simulink model "sldemo_counters_2018a"  (R2018a)
settings: Solver=VariableStepAuto  StartTime=0.0  StopTime=600  FixedStep=.01  RelTol=1e-3  AbsTol=1e-6  EnableMultiTasking=on
libraries: simulink x3
Description:
  | Counters Using Conditionally Executed Subsystems
  | 
  | This model shows the contrast between enabled subsystems and triggered
  | subsystems for the same control signal, through the use of counter circuits.
  | After running the simulation, the scope shows three plots.
  | 
  | The first of these plots shows the control signal which is the output of the discrete
  | pulse generator.
  | 
  | The second plot shows the output of the counter circuit in the enabled subsystem.
  | The counter increments while the subsystem is enabled and then holds its output when
  | the subsystem is disabled. The counter resets to zero when the subsystem is re-enabled
  | because the enable port was configured to reset states when enabling.
  | 
  | The third plot shows the output of the counter circuit in the triggered subsystem. The
  | counter increments every rising edge of the control signal.
  | 
  | The signals are shown in a Signal Viewer scope that does not require a scope block to
  | be put into the block diagram.  Instead, the "scope" icon notation on the ports show
  | that a Signal Viewer is attached.  Double click on the scope icon to make the Signal
  | Viewer appear if it is hidden.
settings Model: ModifiedByFormat=The MathWorks, Inc.  EnablePacing=on  PacingRate=30  ExtModeTrigMode=oneshot  ExtModeArmWhenConnect=off  ExtModeAutoUpdateStatusClock=off  Creator=The MathWorks, Inc.  LastModifiedBy=The MathWorks, Inc.
settings SolverCC: AutoScaleAbsTol=off
settings DataIOCC: SaveFormat=Array
settings OptimizationCC: BlockReduction=off  BooleanDataType=off  ExpressionDepthLimit=2147483647  InitFltsAndDblsToZero=on  LifeSpan=inf  BufferReusableBoundary=off
settings DebuggingCC: SaveWithParameterizedLinksMsg=none  SignalResolutionControl=TryResolveAllWithWarning  MultiTaskDSMMsg=warning  MultiTaskCondExecSysMsg=none  IntegerOverflowMsg=none  FcnCallInpInsideContextMsg=warning  BusObjectLabelMismatch=none  StateNameClashWarn=warning  SFUnexpectedBacktrackingDiag=warning  SFNoUnconditionalDefaultTransitionDiag=warning  SFExecutionAtInitializationDiag=none  IntegerSaturationMsg=none
settings HardwareCC: ProdBitPerPointer=32  ProdBitPerSizeT=32  ProdBitPerPtrDiffT=32  ProdLargestAtomicFloat=None  ProdIntDivRoundTo=Undefined  ProdEndianess=Unspecified  ProdWordSize=32  ProdHWDeviceType=32-bit Generic  TargetUnknown=on
settings ModelReferenceCC: PropagateSignalLabelsOutOfModel=off
settings CodeAppCC: StateflowObjectComments=on
settings GRTTargetCC: TargetFcnLib=ansi_tfl_tmw.mat  TargetLangStandard=C89/C90 (ANSI)  CombineOutputUpdateFcns=off  GRTInterface=on
settings ConfigComp: CovMetricSettings=dw  CovSaveCumulativeToWorkspaceVar=on  CovSaveSingleToWorkspaceVar=on  CovExternalEMLEnable=off  CovSFcnEnable=off

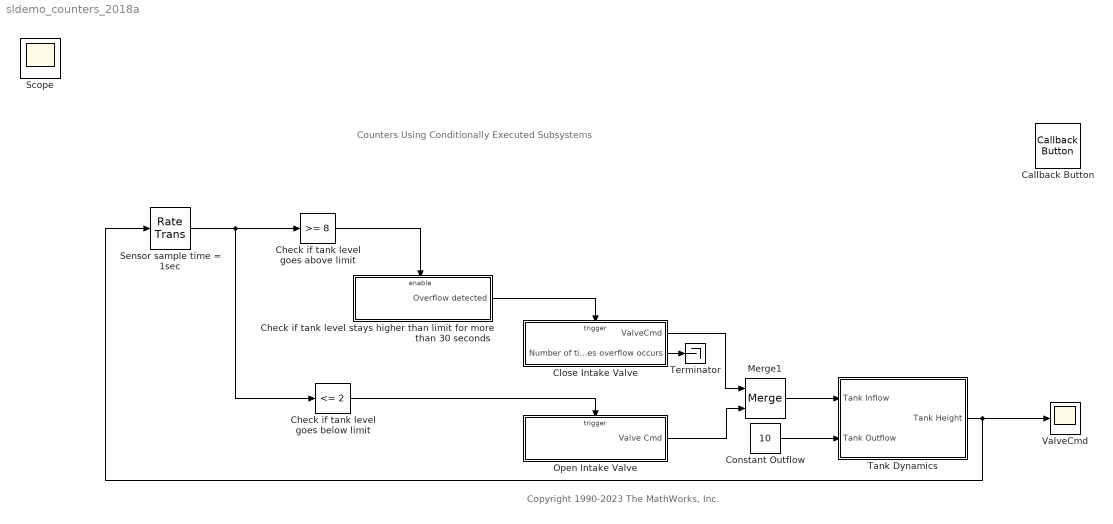
== system sldemo_counters_2018a ==
  note: Counters Using Conditionally Executed Subsystems
  note: Copyright 1990-2023 The MathWorks, Inc.
  Callback Button : CallbackButton  WebBlockId=135  ButtonText=?
      settings: ClickFcn=openExample('simulink_general/sldemo_countersExample')
  Check if tank level goes above limit : simulink/Logic and Bit Operations/Compare To Constant  relop=>=  const=8  OutDataTypeStr=boolean
  Check if tank level goes below limit : simulink/Logic and Bit Operations/Compare To Constant  relop=<=  const=2  OutDataTypeStr=boolean
  Check if tank level stays higher than limit for more than 30 seconds : Subsystem  TreatAsAtomicUnit=on
  Close Intake Valve : Subsystem  TreatAsAtomicUnit=on
  Constant Outflow : Constant  Value=10
  Merge1 : Merge  InitialOutput=2
  Open Intake Valve : Subsystem  TreatAsAtomicUnit=on
  Sensor sample time = 1sec : RateTransition  OutPortSampleTime=1
  Tank Dynamics : Subsystem
  Terminator : Terminator
  ValveCmd : Scope
  Scope : Scope
  wires:
  Close Intake Valve/1(ValveCmd) -> Merge1/1
  Constant Outflow/1 -> Tank Dynamics/2(Tank Outflow)
  Open Intake Valve/1(Valve Cmd) -> Merge1/2
  Check if tank level goes below limit/1 -> Open Intake Valve/Trigger
  Check if tank level stays higher than limit for more than 30 seconds/1(Overflow detected) -> Close Intake Valve/Trigger
  Merge1/1 -> Tank Dynamics/1(Tank Inflow)
  Close Intake Valve/2(Number of times overflow occurs) -> Terminator/1
  Sensor sample time = 1sec/1 -> Check if tank level goes above limit/1, Check if tank level goes below limit/1
  Tank Dynamics/1(Tank Height) -> Sensor sample time = 1sec/1, ValveCmd/1
  Check if tank level goes above limit/1 -> Check if tank level stays higher than limit for more than 30 seconds/Enable

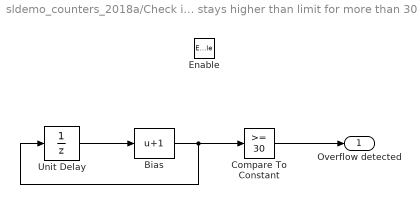
== system sldemo_counters_2018a/Check if tank level stays higher than limit for more than 30 seconds ==
  Enable : EnablePort  StatesWhenEnabling=reset
  Bias : Bias  Bias=1
  Compare To Constant : simulink/Logic and Bit Operations/Compare To Constant  relop=>=  const=30  OutDataTypeStr=boolean
  Unit Delay : UnitDelay  SampleTime=-1
  Overflow detected : Outport  VectorParamsAs1DForOutWhenUnconnected=on
  wires:
  Unit Delay/1 -> Bias/1
  Bias/1 -> Compare To Constant/1, Unit Delay/1
  Compare To Constant/1 -> Overflow detected/1

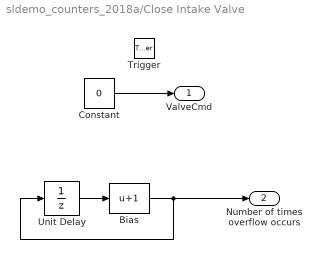
== system sldemo_counters_2018a/Close Intake Valve ==
  Trigger : TriggerPort  VariantControl=(inherit)
  Bias : Bias  Bias=1
  Constant : Constant  Value=0  SampleTime=-1
  Unit Delay : UnitDelay  SampleTime=-1
  ValveCmd : Outport  VectorParamsAs1DForOutWhenUnconnected=on
  Number of times overflow occurs : Outport  Port=2  VectorParamsAs1DForOutWhenUnconnected=on
  wires:
  Constant/1 -> ValveCmd/1
  Unit Delay/1 -> Bias/1
  Bias/1 -> Number of times overflow occurs/1, Unit Delay/1

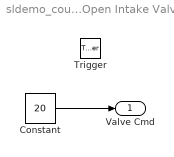
== system sldemo_counters_2018a/Open Intake Valve ==
  Trigger : TriggerPort  VariantControl=(inherit)
  Constant : Constant  Value=20  SampleTime=-1
  Valve Cmd : Outport  InitialOutput=0  VectorParamsAs1DForOutWhenUnconnected=on
  wires:
  Constant/1 -> Valve Cmd/1

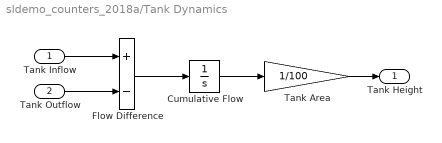
== system sldemo_counters_2018a/Tank Dynamics ==
  Tank Inflow : Inport
  Tank Outflow : Inport  Port=2
  Cumulative Flow : Integrator  InitialCondition=500
  Flow Difference : Sum  Inputs=+-  SaturateOnIntegerOverflow=on  InputSameDT=on  OutDataTypeStr=Inherit: Same as first input
  Tank Area : Gain  Gain=1/100  SaturateOnIntegerOverflow=on  OutDataTypeStr=Inherit: Same as input  ParamDataTypeStr=Inherit: Same as input
  Tank Height : Outport  InitialOutput=0
  wires:
  Tank Outflow/1 -> Flow Difference/2
  Tank Inflow/1 -> Flow Difference/1
  Flow Difference/1 -> Cumulative Flow/1
  Cumulative Flow/1 -> Tank Area/1
  Tank Area/1 -> Tank Height/1
